simulink model "req7"  (R2019a)
settings: Solver=FixedStepAuto  StartTime=0.0  StopTime=100  RelTol=1e-3
settings Model: Creator=e40014285  LastModifiedBy=e40014285
settings ConfigComp: CovEnable=on  CovScope=ReferencedModels  RecordCoverage=on

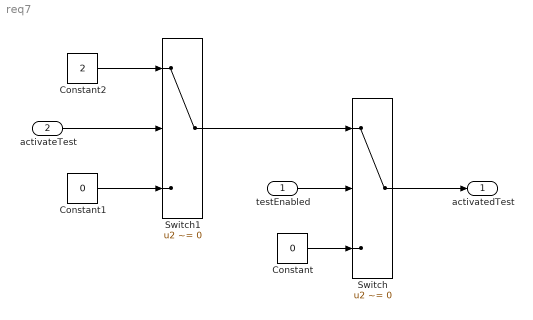
== system req7 ==
  testEnabled : Inport
  activateTest : Inport  Port=2
  Constant : Constant  Value=0
  Constant1 : Constant  Value=0
  Constant2 : Constant  Value=2
  Switch : Switch  Criteria=u2 ~= 0  Threshold=~0
  Switch1 : Switch  Criteria=u2 ~= 0  Threshold=~0
  activatedTest : Outport
  wires:
  Switch1/1 -> Switch/1
  Switch/1 -> activatedTest/1
  testEnabled/1 -> Switch/2
  Constant/1 -> Switch/3
  activateTest/1 -> Switch1/2
  Constant1/1 -> Switch1/3
  Constant2/1 -> Switch1/1
